simulink model "controller_dev"  (R2018b)
settings: Solver=ode2  StartTime=0.0  StopTime=200  FixedStep=0.002  RelTol=1e-3  EnableMultiTasking=on
model workspace (MAT data in the model file):
  m = 1000
settings Model: DataDictionary=controller_dev.sldd  PauseTimes=9.280  Creator=wischnewski  LastModifiedBy=ga25xiw
settings DataIOCC: SaveFormat=StructureWithTime
settings OptimizationCC: BlockReduction=off  DefaultParameterBehavior=Inlined  OptimizeBlockIOStorage=off  BufferReuse=off  GlobalBufferReuse=off  ExpressionFolding=off  LocalBlockOutputs=off  LifeSpan=inf  OptimizeDataStoreBuffers=off  BusAssignmentInplaceUpdate=off
settings HardwareCC: ProdBitPerPointer=32  ProdBitPerSizeT=32  ProdBitPerPtrDiffT=32  ProdLargestAtomicFloat=None  ProdWordSize=32  ProdLongLongMode=on  ProdHWDeviceType=Generic->32-bit x86 compatible
settings ModelReferenceCC: ModelReferenceMinAlgLoopOccurrences=on
settings SFSimCC: SimUseLocalCustomCode=off
settings RTWCC: Description=Generic Real-Time Target  GenerateReport=on  RTWUseLocalCustomCode=off  LaunchReport=on
settings CodeAppCC: ForceParamTrailComments=on  OperatorAnnotations=on  StateflowObjectComments=on  MATLABSourceComments=on
settings GRTTargetCC: TargetLangStandard=C89/C90 (ANSI)

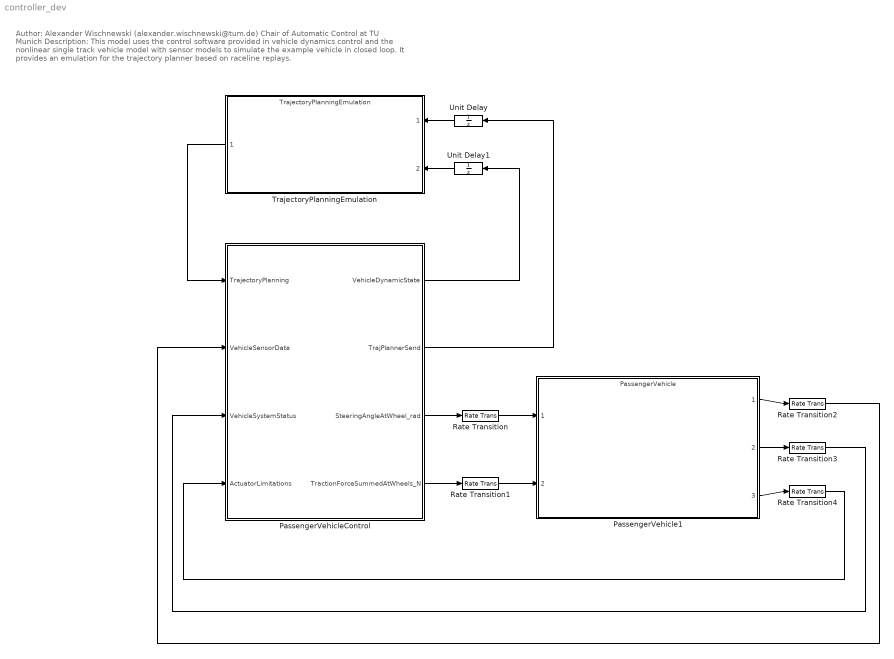
== system controller_dev ==
  note: Author: Alexander Wischnewski (alexander.wischnewski@tum.de)
      | Chair of Automatic Control at TU Munich
      |
      | Description: This model uses the control software provided in vehicle dynamics control and the nonlinear single track vehicle model
      | with sensor models to simulate the example vehicle in closed loop. It provides an emulation for the trajectory planner based on raceline replays.
  PassengerVehicle1 : ModelReference  ModelNameDialog=PassengerVehicle  SimulationMode=Normal  ModelReferenceVersion=1.716
  PassengerVehicleControl : Subsystem
  Rate Transition{,1..4} (5 alike) : RateTransition
  TrajectoryPlanningEmulation : ModelReference  ModelNameDialog=TrajectoryPlanningEmulation.slx  ParameterArgumentNames=Raceline  ParameterArgumentValues=Raceline  UsingDefaultArgumentValue=0  SimulationMode=Normal  ModelReferenceVersion=1.703
  Unit Delay : UnitDelay  SampleTime=-1
  Unit Delay1 : UnitDelay  SampleTime=-1
  wires:
  PassengerVehicleControl/3(SteeringAngleAtWheel_rad) -> Rate Transition/1
  PassengerVehicleControl/4(TractionForceSummedAtWheels_N) -> Rate Transition1/1
  TrajectoryPlanningEmulation/1 -> PassengerVehicleControl/1(TrajectoryPlanning)
  PassengerVehicleControl/1(VehicleDynamicState) -> Unit Delay1/1
  PassengerVehicleControl/2(TrajPlannerSend) -> Unit Delay/1
  Unit Delay/1 -> TrajectoryPlanningEmulation/1
  Unit Delay1/1 -> TrajectoryPlanningEmulation/2
  PassengerVehicle1/3 -> Rate Transition4/1
  Rate Transition4/1 -> PassengerVehicleControl/4(ActuatorLimitations)
  PassengerVehicle1/2 -> Rate Transition3/1
  Rate Transition3/1 -> PassengerVehicleControl/3(VehicleSystemStatus)
  PassengerVehicle1/1 -> Rate Transition2/1
  Rate Transition2/1 -> PassengerVehicleControl/2(VehicleSensorData)
  Rate Transition/1 -> PassengerVehicle1/1
  Rate Transition1/1 -> PassengerVehicle1/2

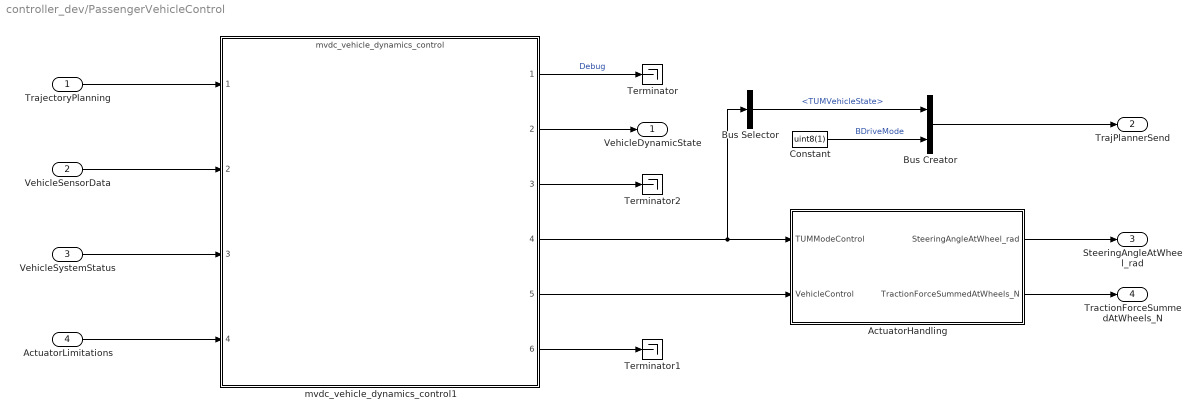
== system controller_dev/PassengerVehicleControl ==
  TrajectoryPlanning : Inport
  VehicleSensorData : Inport  Port=2
  VehicleSystemStatus : Inport  Port=3
  ActuatorLimitations : Inport  Port=4
  ActuatorHandling : Subsystem
  Bus Creator : BusCreator  Inputs=2
  Bus Selector : BusSelector  OutputSignals=TUMVehicleState
  Constant : Constant  Value=uint8(1)
  Terminator : Terminator
  Terminator1 : Terminator
  Terminator2 : Terminator
  mvdc_vehicle_dynamics_control1 : ModelReference  ModelNameDialog=mvdc_vehicle_dynamics_control  SimulationMode=Normal  ModelReferenceVersion=1.757
  VehicleDynamicState : Outport
  TrajPlannerSend : Outport  Port=2
  SteeringAngleAtWheel_rad : Outport  Port=3
  TractionForceSummedAtWheels_N : Outport  Port=4
  wires:
  mvdc_vehicle_dynamics_control1/1 -> Terminator/1  "Debug"
  VehicleSystemStatus/1 -> mvdc_vehicle_dynamics_control1/3
  ActuatorLimitations/1 -> mvdc_vehicle_dynamics_control1/4
  VehicleSensorData/1 -> mvdc_vehicle_dynamics_control1/2
  TrajectoryPlanning/1 -> mvdc_vehicle_dynamics_control1/1
  mvdc_vehicle_dynamics_control1/5 -> ActuatorHandling/2(VehicleControl)
  mvdc_vehicle_dynamics_control1/4 -> Bus Selector/1, ActuatorHandling/1(TUMModeControl)
  mvdc_vehicle_dynamics_control1/6 -> Terminator1/1
  mvdc_vehicle_dynamics_control1/3 -> Terminator2/1
  mvdc_vehicle_dynamics_control1/2 -> VehicleDynamicState/1
  ActuatorHandling/2(TractionForceSummedAtWheels_N) -> TractionForceSummedAtWheels_N/1
  ActuatorHandling/1(SteeringAngleAtWheel_rad) -> SteeringAngleAtWheel_rad/1
  Bus Selector/1 -> Bus Creator/1  "<TUMVehicleState>"
  Constant/1 -> Bus Creator/2  "BDriveMode"
  Bus Creator/1 -> TrajPlannerSend/1

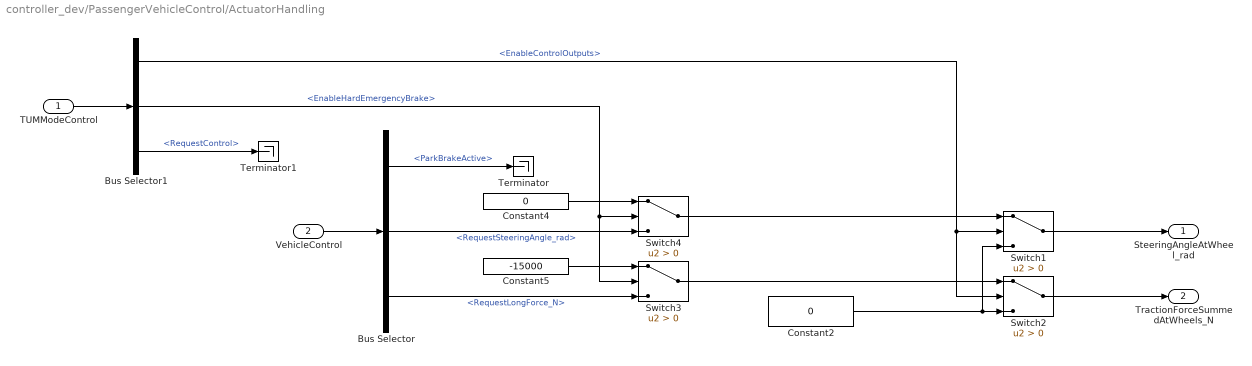
== system controller_dev/PassengerVehicleControl/ActuatorHandling ==
  TUMModeControl : Inport  OutDataTypeStr=Bus: TUMModeControl
  VehicleControl : Inport  Port=2  OutDataTypeStr=Bus: VehicleControl
  Bus Selector : BusSelector  OutputSignals=ParkBrakeActive,RequestSteeringAngle_rad,RequestLongForce_N
  Bus Selector1 : BusSelector  OutputSignals=EnableControlOutputs,EnableHardEmergencyBrake,RequestControl
  Constant2 : Constant  Value=0
  Constant4 : Constant  Value=0
  Constant5 : Constant  Value=-15000
  Switch{1..4} (4 alike) : Switch  Criteria=u2 > Threshold
  Terminator : Terminator
  Terminator1 : Terminator
  SteeringAngleAtWheel_rad : Outport
  TractionForceSummedAtWheels_N : Outport  Port=2
  wires:
  Bus Selector1/1 -> Switch2/2, Switch1/2  "<EnableControlOutputs>"
  TUMModeControl/1 -> Bus Selector1/1
  Bus Selector/3 -> Switch3/3  "<RequestLongForce_N>"
  Constant2/1 -> Switch1/3, Switch2/3
  VehicleControl/1 -> Bus Selector/1
  Bus Selector/2 -> Switch4/3  "<RequestSteeringAngle_rad>"
  Constant4/1 -> Switch4/1
  Constant5/1 -> Switch3/1
  Bus Selector1/2 -> Switch3/2, Switch4/2  "<EnableHardEmergencyBrake>"
  Bus Selector/1 -> Terminator/1  "<ParkBrakeActive>"
  Bus Selector1/3 -> Terminator1/1  "<RequestControl>"
  Switch4/1 -> Switch1/1
  Switch3/1 -> Switch2/1
  Switch1/1 -> SteeringAngleAtWheel_rad/1
  Switch2/1 -> TractionForceSummedAtWheels_N/1
